simulink model "simulinkmodel"  (R2025a)
settings: Solver=VariableStepAuto  StartTime=0.0  StopTime=800  RelTol=1e-3
undefined symbols (not defined in the file): A01, A02, At1, At2, g, Kp
settings Model: Creator=LENOVO  LastModifiedBy=LENOVO

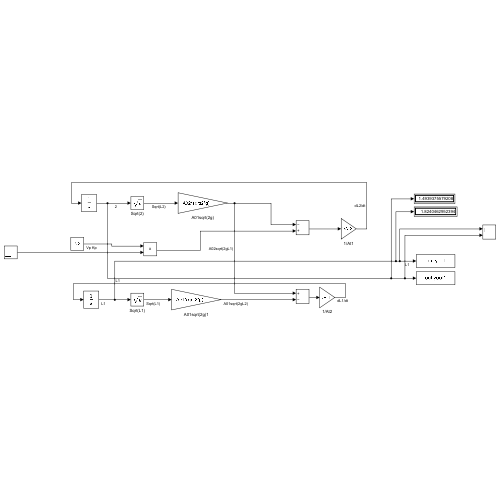
[thumbnail: Simulink's stored preview of the top-level diagram]
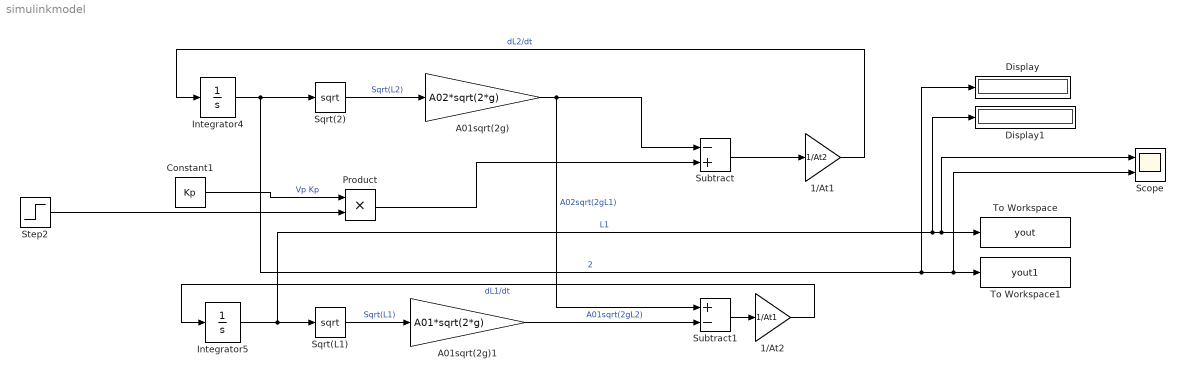
== system simulinkmodel ==
  1/At1 : Gain  Gain=1/At2
  1/At2 : Gain  Gain=1/At1
  A01sqrt(2g) : Gain  Gain=A02*sqrt(2*g)
  A01sqrt(2g)1 : Gain  Gain=A01*sqrt(2*g)
  Constant1 : Constant  Value=Kp
  Display : Display
  Display1 : Display
  Integrator4 : Integrator
  Integrator5 : Integrator
  Product : Product
  Scope : Scope  NumInputPorts=2
      settings: ActiveDisplayYMinimum=-1  ActiveDisplayYMaximum=1
  Sqrt(2) : Sqrt
  Sqrt(L1) : Sqrt
  Step2 : Step  Time=0  After=5
  Subtract : Sum  Inputs=-+
  Subtract1 : Sum  Inputs=+-
  To Workspace : ToWorkspace  VariableName=yout  SaveFormat=Structure With Time  SampleTime=-1
  To Workspace1 : ToWorkspace  VariableName=yout1  SaveFormat=Structure With Time  SampleTime=-1
  wires:
  1/At1/1 -> Integrator4/1  "dL2/dt"
  Integrator4/1 -> Display/1, Scope/2, To Workspace1/1, Sqrt(2)/1  "2"
  Subtract1/1 -> 1/At2/1
  A01sqrt(2g)/1 -> Subtract1/1, Subtract/1  "A02sqrt(2gL1)"
  Product/1 -> Subtract/2
  Subtract/1 -> 1/At1/1
  Integrator5/1 -> Display1/1, Scope/1, To Workspace/1, Sqrt(L1)/1  "L1"
  Constant1/1 -> Product/1  "Vp Kp"
  A01sqrt(2g)1/1 -> Subtract1/2  "A01sqrt(2gL2)"
  Sqrt(2)/1 -> A01sqrt(2g)/1  "Sqrt(L2)"
  Sqrt(L1)/1 -> A01sqrt(2g)1/1  "Sqrt(L1)"
  Step2/1 -> Product/2
  1/At2/1 -> Integrator5/1  "dL1/dt"
